simulink model "FBsimDC_closed"  (R2018b)
settings: Solver=ode4  StartTime=0.0  StopTime=0.5e-3*0+0.5*1+0.8*0  FixedStep=Tsim  MaxStep=1e-4  RelTol=1e-6
PreLoadFcn:
  | uC=Simulink.Signal;
  | uC.RTWInfo.STorageClass='ExportedGlobal';
  | uC.InitialValue='0.5';
undefined symbols (not defined in the file): C1, C3, fsw, imax, J, Ke, kiI, kiMR, kiW, kpI, kpMR, kpW, Kt, La, Ra, Ts, Tsim, Tsm, Tw, Vdc, wmax
libraries: powerlib x11, simulink x7, powerlib_meascontrol x1, peGeneralControl x1
settings Model: Creator=matti  LastModifiedBy=matti
settings DataIOCC: ReturnWorkspaceOutputs=on

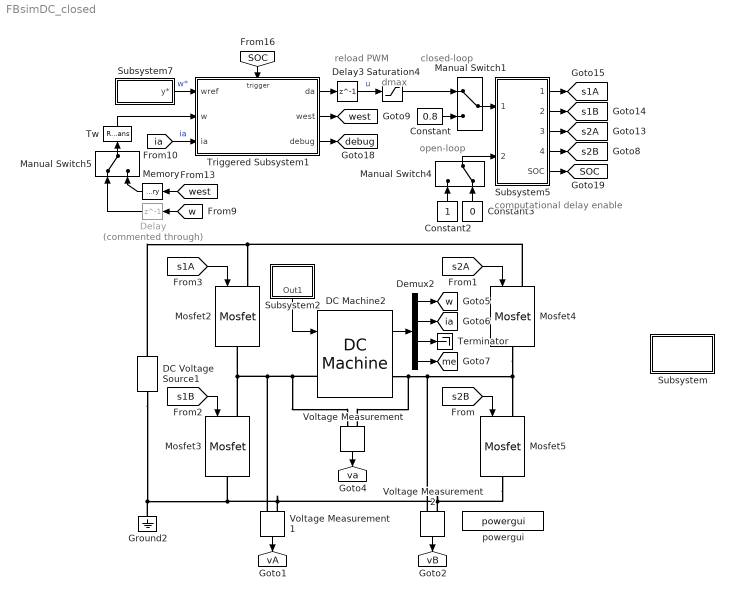
== system FBsimDC_closed ==
  note: closed-loop
  note: open-loop
  note: reload
      | PWM
  note: computational delay
      | enable
  note: dmax
  Constant : Constant  Value=0.8  SampleTime=Ts
  Constant2 : Constant  SampleTime=Ts
  Constant3 : Constant  Value=0  SampleTime=Ts
  DC Machine2 : powerlib/Machines/DC Machine  PresetModel=No  MechanicalLoad=Torque TL  FieldType=Permanent magnet  ShowDetailedParameters=on  MeasurementBus=off  RLa="[Ra  La]"  RLf="[ 240  120]"  Laf=1.8  MachineConstant=Torque constant (N.m/A)  Ke=1.8  Kt=Kt  J=J  Bm=B  Tf=0  w0=0  Ifinit=1  TsPowergui=0  TsBlock=-1
      settings: SourceProductName=Simscape Electrical
  DC Voltage Source1 : powerlib/Electrical Sources/DC Voltage Source  Amplitude=Vdc  Measurements=None
      settings: SourceProductName=Simscape Electrical
  Delay : Delay  Commented=through  DelayLength=1  SampleTime=Tw
  Delay3 : Delay  DelayLength=1  InitialCondition=0.5  SampleTime=Ts/2
  Demux2 : Demux  BusSelectionMode=on
  Ground2 : powerlib/Elements/Ground  LConnTagsString=a
      settings: SourceProductName=Simscape Electrical
  Manual Switch1 : ManualSwitch
  Manual Switch4 : ManualSwitch  CurrentSetting=0
  Manual Switch5 : ManualSwitch
  Memory : Memory  InheritSampleTime=on
  Mosfet{2..5} (4 alike) : powerlib/Power Electronics/Mosfet  Ron=0.1  Lon=0  Rd=0.01  Vfd=0  IC=0  Rs=1e5  Cs=inf  Measurements=off
      settings: SourceProductName=Simscape Electrical
  Saturation4 : Saturate  UpperLimit=1  LowerLimit=0
  Subsystem : Subsystem
      mask Display: disp('stream')
  Subsystem2 : Subsystem
      mask Display: disp('load\ntorque')
  Subsystem5 : Subsystem
      mask Display: disp('modulator')
  Subsystem7 : Subsystem
      mask Display: disp('reference')
  Terminator : Terminator
  Triggered Subsystem1 : Subsystem  TreatAsAtomicUnit=on
      mask Display: disp('cascade controller\n(syncronized with PWM)')
  Tw : RateTransition  OutPortSampleTime=Tw
  Voltage Measurement : powerlib/Measurements/Voltage Measurement  PhasorSimulation=off  OutputType=Complex  PSBequivalent=0
  Voltage Measurement1 : powerlib/Measurements/Voltage Measurement  PhasorSimulation=off  OutputType=Complex  PSBequivalent=0
  Voltage Measurement2 : powerlib/Measurements/Voltage Measurement  PhasorSimulation=off  OutputType=Complex  PSBequivalent=0
  powergui : powerlib/powergui  Priority=1  SimulationMode=Continuous  SampleTime=1/(400*fsw)  frequency=60  Iterations=50  frequencyindice=0  Pbase=100e6  ErrMax=1e-4  UnitsV=kV  UnitsW=MW  buscounter=0  FunctionMessages=on  echomessages=off  EnableUseOfTLC=off  CurrentSourceSwitches=off  DisableSnubberDevices=on  DisableRonSwitches=on  DisableVfSwitches=on  DisplayEquations=off  SolverType=Tustin/Backward Euler (TBE)  Interpol=off  ExternalGateDelay=off  methode=off  Ts=100  x0status=blocks  SPID=off  SwTol=0  HookPort=off  RestoreLinks=warning  ResistiveCurrentMeasurement=off  Frange=[0:2:500]  Ylog=off  Xlog=on  ShowGrid=off  save=off  variable=ZData  structure=0  ZoomFFT=off  StartTime=0.0  cycles=1  DisplayStyle=1  fundamental=60  FreqAxis=off  MaxFrequency=1000  frequencyindicesteady=1  RmsSteady=1  display=off
  tag scope: SOC=global, debug=global, ia=global, me=global, s1A=global, s1B=global, s2A=global, s2B=global, vA=global, vB=global, va=global, w=global, west=global
  wires:
  DC Machine2/1 -> Demux2/1
  [s2B] -> Mosfet5/1
  [s2A] -> Mosfet4/1
  [s1B] -> Mosfet3/1
  [s1A] -> Mosfet2/1
  Demux2/3 -> Terminator/1
  Voltage Measurement/1 -> [va]
  Demux2/1 -> [w]
  Demux2/2 -> [ia]
  Demux2/4 -> [me]
  Subsystem5/3(Out3) -> [s2A]
  Subsystem5/1(Out1) -> [s1A]
  Subsystem5/4(Out4) -> [s2B]
  Subsystem5/2(Out2) -> [s1B]
  Manual Switch1/1 -> Subsystem5/1(modA)
  Saturation4/1 -> Manual Switch1/1
  Constant/1 -> Manual Switch1/2
  Subsystem2/1(Out1) -> DC Machine2/1
  [west] -> Memory/1
  Triggered Subsystem1/1(da) -> Delay3/1
  Manual Switch5/1 -> Tw/1
  [SOC] -> Triggered Subsystem1/Trigger
  Constant3/1 -> Manual Switch4/2
  Subsystem7/1(y*) -> Triggered Subsystem1/1(wref)  "w*"
  Delay3/1 -> Saturation4/1  "u"
  Triggered Subsystem1/3(debug) -> [debug]
  Constant2/1 -> Manual Switch4/1
  Manual Switch4/1 -> Subsystem5/2(enable delay)
  Subsystem5/5(SOC) -> [SOC]
  [ia] -> Triggered Subsystem1/3(ia)  "ia"
  Triggered Subsystem1/2(west) -> [west]
  Memory/1 -> Manual Switch5/2
  Voltage Measurement1/1 -> [vA]
  Voltage Measurement2/1 -> [vB]
  Tw/1 -> Triggered Subsystem1/2(w)
  [w] -> Delay/1
  Delay/1 -> Manual Switch5/1
  connections:
  Mosfet3/RConn1 -- Voltage Measurement2/LConn2 -- Mosfet5/RConn1 -- Voltage Measurement1/LConn2 -- Ground2/LConn1 -- DC Voltage Source1/LConn1
  Mosfet4/LConn1 -- DC Voltage Source1/RConn1 -- Mosfet2/LConn1
  Mosfet4/RConn1 -- Voltage Measurement2/LConn1 -- Voltage Measurement/LConn2 -- DC Machine2/RConn1 -- Mosfet5/LConn1
  Mosfet3/LConn1 -- Voltage Measurement1/LConn1 -- DC Machine2/LConn1 -- Voltage Measurement/LConn1 -- Mosfet2/RConn1

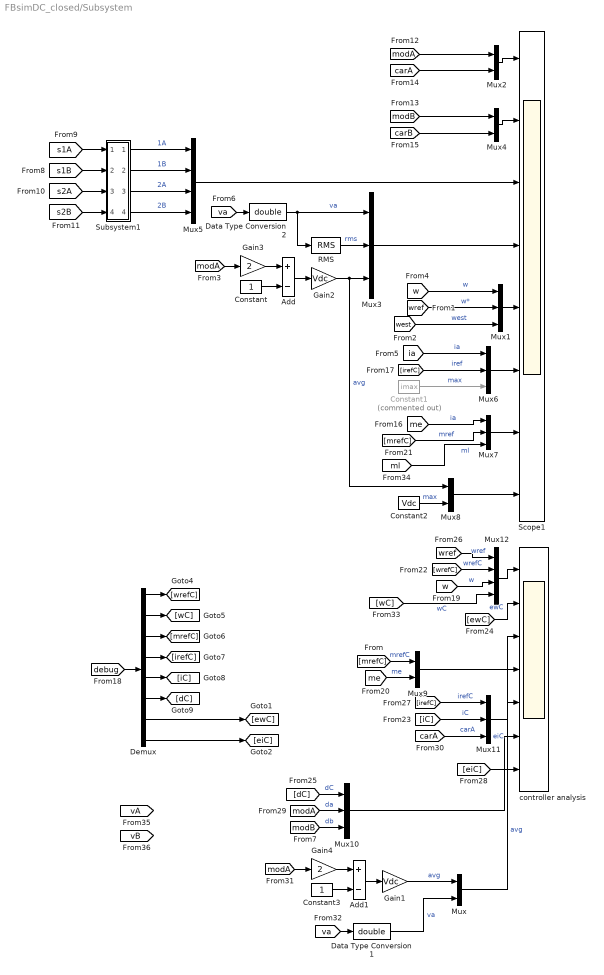
== system FBsimDC_closed/Subsystem ==
  Add : Sum  Inputs=+-
  Add1 : Sum  Inputs=+-
  Constant : Constant  SampleTime=Ts
  Constant1 : Constant  Commented=on  Value=imax  SampleTime=Ts
  Constant2 : Constant  Value=Vdc  SampleTime=Ts
  Constant3 : Constant  SampleTime=Ts
  Data Type Conversion1 : DataTypeConversion  OutDataTypeStr=double
  Data Type Conversion2 : DataTypeConversion  OutDataTypeStr=double
  Demux : Demux  Outputs=8
  Gain1 : Gain  Gain=Vdc
  Gain2 : Gain  Gain=Vdc
  Gain3 : Gain  Gain=2
  Gain4 : Gain  Gain=2
  Mux{,2,4,8..9} (5 alike) : Mux  Inputs=2
  Mux{1,3,6..7,10..11} (6 alike) : Mux  Inputs=3
  Mux12 : Mux
  Mux5 : Mux
  RMS : powerlib_meascontrol/Measurements/RMS  TrueRMS=on  Freq=fsw  RMSInit=0  Ts=0
  Scope1 : Scope  NumInputPorts=8
  Subsystem1 : Subsystem
      mask Display: disp('shift')
  controller analysis : Scope  NumInputPorts=7
  wires:
  [modA] -> Mux2/1
  Mux3/1 -> Scope1/4
  [s2B] -> Subsystem1/4(In4)
  [carA] -> Mux2/2
  [s1A] -> Subsystem1/1(In1)
  [va] -> Data Type Conversion2/1
  Mux2/1 -> Scope1/1
  [s2A] -> Subsystem1/3(In3)
  Mux4/1 -> Scope1/2
  [modB] -> Mux4/1
  Data Type Conversion2/1 -> Mux3/1, RMS/1  "va"
  [s1B] -> Subsystem1/2(In2)
  [carB] -> Mux4/2
  Subsystem1/3(Out3) -> Mux5/3  "2A"
  Subsystem1/4(Out4) -> Mux5/4  "2B"
  Subsystem1/2(Out2) -> Mux5/2  "1B"
  Subsystem1/1(Out1) -> Mux5/1  "1A"
  Mux5/1 -> Scope1/3
  Gain3/1 -> Add/1
  Gain2/1 -> Mux3/3, Mux8/1  "avg"
  Constant/1 -> Add/2
  [modA] -> Gain3/1
  Add/1 -> Gain2/1
  RMS/1 -> Mux3/2  "rms"
  [irefC] -> Mux6/2  "iref"
  [ia] -> Mux6/1  "ia"
  Mux6/1 -> Scope1/6
  [wref] -> Mux1/2  "w*"
  [w] -> Mux1/1  "w"
  Mux1/1 -> Scope1/5
  Mux7/1 -> Scope1/7
  [me] -> Mux7/1  "ia"
  [mrefC] -> Mux7/2  "mref"
  Constant1/1 -> Mux6/3  "max"
  Mux8/1 -> Scope1/8
  Constant2/1 -> Mux8/2  "max"
  [west] -> Mux1/3  "west"
  [debug] -> Demux/1
  Mux11/1 -> controller analysis/4
  [carA] -> Mux11/3  "carA"
  [dC] -> Mux10/1  "dC"
  [wrefC] -> Mux12/2  "wrefC"
  [modA] -> Mux10/2  "da"
  [irefC] -> Mux11/1  "irefC"
  Mux12/1 -> controller analysis/1
  [iC] -> Mux11/2  "iC"
  [wref] -> Mux12/1  "wref"
  Mux10/1 -> controller analysis/6
  Demux/1 -> [wrefC]
  Demux/2 -> [wC]
  Demux/3 -> [mrefC]
  Demux/4 -> [irefC]
  Demux/5 -> [iC]
  Demux/6 -> [dC]
  [w] -> Mux12/3  "w"
  Mux9/1 -> controller analysis/3
  [mrefC] -> Mux9/1  "mrefC"
  [me] -> Mux9/2  "me"
  [modB] -> Mux10/3  "db"
  [ewC] -> controller analysis/2  "ewC"
  Demux/7 -> [ewC]
  Demux/8 -> [eiC]
  [eiC] -> controller analysis/5  "eiC"
  Add1/1 -> Gain1/1
  [modA] -> Gain4/1
  Constant3/1 -> Add1/2
  Gain4/1 -> Add1/1
  Mux/1 -> controller analysis/7  "avg"
  [va] -> Data Type Conversion1/1
  Gain1/1 -> Mux/1  "avg"
  Data Type Conversion1/1 -> Mux/2  "va"
  [wC] -> Mux12/4  "wC"
  [ml] -> Mux7/3  "ml"

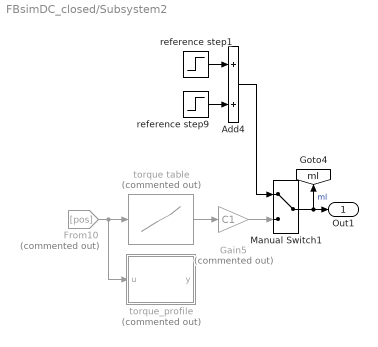
== system FBsimDC_closed/Subsystem2 ==
  Add4 : Sum
  From10 : From  Commented=on  GotoTag=pos  TagVisibility=global
  Gain5 : Gain  Commented=on  Gain=C1
  Manual Switch1 : ManualSwitch
  reference step1 : Step  Time=0.1  After=0.03  SampleTime=Ts
  reference step9 : Step  Time=0.3  After=-0.03  SampleTime=Ts
  torque table : Lookup_n-D  Commented=on  NumberOfTableDimensions=1  BreakpointsForDimension1=[0 1 3 4 6 8 9 10]  Table=[ 0, 0, 26000*9.81*sin(atan(5/100)), 0, 0, 26000*9.81*sin(atan(-5/100)), 0 0]  InterpMethod=Flat  InternalRulePriority=Speed  RndMeth=Simplest  InputSameDT=on
  torque_profile : MATLAB Function  Commented=on  TreatAsAtomicUnit=on
  Out1 : Outport
  tag scope: ml=global
  wires:
  Manual Switch1/1 -> [ml], Out1/1  "ml"
  torque table/1 -> Gain5/1
  From10/1 -> torque_profile/1(u), torque table/1
  Gain5/1 -> Manual Switch1/2
  reference step9/1 -> Add4/2
  Add4/1 -> Manual Switch1/1
  reference step1/1 -> Add4/1

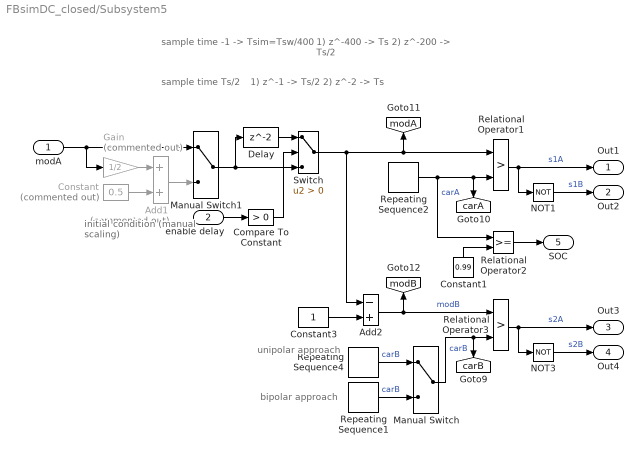
== system FBsimDC_closed/Subsystem5 ==
  note: initial condition
      | (manual scaling)
  note: unipolar approach
  note: bipolar approach
  note: sample time Ts/2
  note: sample time -1 -> Tsim=Tsw/400
  note: 1)  z^-1 -> Ts/2
      | 2)  z^-2 -> Ts
  note: 1)  z^-400 -> Ts
      | 2)  z^-200 -> Ts/2
  modA : Inport
  enable delay : Inport  Port=2
  Add1 : Sum  Commented=on
  Add2 : Sum  Inputs=-+
  Compare To Constant : simulink/Logic and Bit Operations/Compare To Constant  relop=>  const=0  OutDataTypeStr=boolean
  Constant : Constant  Commented=on  Value=0.5  SampleTime=Ts
  Constant1 : Constant  Value=0.99  SampleTime=Ts
  Constant3 : Constant  SampleTime=Ts
  Delay : Delay  SampleTime=Ts
  Gain : Gain  Commented=on  Gain=1/2
  Manual Switch : ManualSwitch
  Manual Switch1 : ManualSwitch
  NOT1 : Logic  Operator=NOT  IconShape=distinctive  AllPortsSameDT=off  OutDataTypeStr=boolean
  NOT3 : Logic  Operator=NOT  IconShape=distinctive  AllPortsSameDT=off  OutDataTypeStr=boolean
  Relational Operator1 : RelationalOperator  Operator=>  OutDataTypeStr=boolean  RndMeth=Simplest
  Relational Operator2 : RelationalOperator  OutDataTypeStr=boolean  RndMeth=Simplest
  Relational Operator3 : RelationalOperator  Operator=>  OutDataTypeStr=boolean  RndMeth=Simplest
  Repeating Sequence1 : simulink/Sources/Repeating Sequence  rep_seq_t=[0 1/(2*fsw) 1/fsw]  rep_seq_y=[1 0 1]
  Repeating Sequence2 : simulink/Sources/Repeating Sequence  rep_seq_t=[0 1/(2*fsw) 1/fsw]  rep_seq_y=[0 1 0]
  Repeating Sequence4 : simulink/Sources/Repeating Sequence  rep_seq_t=[0 1/(2*fsw) 1/fsw]  rep_seq_y=[0 1 0]
  Switch : Switch  Criteria=u2 > Threshold
  Out1 : Outport
  Out2 : Outport  Port=2
  Out3 : Outport  Port=3
  Out4 : Outport  Port=4
  SOC : Outport  Port=5
  tag scope: carA=global, carB=global, modA=global, modB=global
  wires:
  Constant3/1 -> Add2/2
  Manual Switch/1 -> [carB], Relational Operator3/2  "carB"
  Add2/1 -> Relational Operator3/1, [modB]  "modB"
  Relational Operator3/1 -> Out3/1, NOT3/1  "s2A"
  Repeating Sequence1/1 -> Manual Switch/2  "carB"
  NOT3/1 -> Out4/1  "s2B"
  Repeating Sequence4/1 -> Manual Switch/1  "carB"
  Relational Operator1/1 -> Out1/1, NOT1/1  "s1A"
  NOT1/1 -> Out2/1  "s1B"
  modA/1 -> Manual Switch1/1, Gain/1
  Constant/1 -> Add1/2
  Add1/1 -> Manual Switch1/2
  Gain/1 -> Add1/1
  Relational Operator2/1 -> SOC/1
  Repeating Sequence2/1 -> Relational Operator2/1, [carA], Relational Operator1/2  "carA"
  Constant1/1 -> Relational Operator2/2
  Switch/1 -> Add2/1, Relational Operator1/1, [modA]
  Compare To Constant/1 -> Switch/2
  Delay/1 -> Switch/1
  enable delay/1 -> Compare To Constant/1
  Manual Switch1/1 -> Delay/1, Switch/3

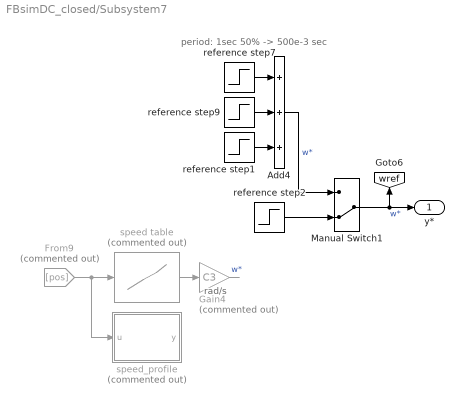
== system FBsimDC_closed/Subsystem7 ==
  note: period: 1sec 50% -> 500e-3 sec
  note: rad/s
  Add4 : Sum  Inputs=+++
  From9 : From  Commented=on  GotoTag=pos
  Gain4 : Gain  Commented=on  Gain=C3
  Manual Switch1 : ManualSwitch  CurrentSetting=0
  reference step1 : Step  Time=0.005+0.15+500e-3  After=200  SampleTime=Ts
  reference step2 : Step  Time=0.005  After=100  SampleTime=Ts
  reference step7 : Step  Time=0.005  After=100  SampleTime=Ts
  reference step9 : Step  Time=0.005+0.15  After=-200  SampleTime=Ts
  speed table : Lookup_n-D  Commented=on  NumberOfTableDimensions=1  BreakpointsForDimension1=[0 1 3 4 6 8 9 10]  Table=[35 60 60 75 60 60 35 0]  InterpMethod=Flat  ExtrapMethod=Clip  UseLastTableValue=on  InternalRulePriority=Speed  RndMeth=Simplest  InputSameDT=on
  speed_profile : MATLAB Function  Commented=on  TreatAsAtomicUnit=on
  y* : Outport
  tag scope: wref=global
  wires:
  Manual Switch1/1 -> [wref], y*/1  "w*"
  Add4/1 -> Manual Switch1/1  "w*"
  From9/1 -> speed_profile/1(u), speed table/1
  speed table/1 -> Gain4/1
  Gain4/1 -> ?  "w*"
  reference step7/1 -> Add4/1
  reference step9/1 -> Add4/2
  reference step1/1 -> Add4/3
  reference step2/1 -> Manual Switch1/2

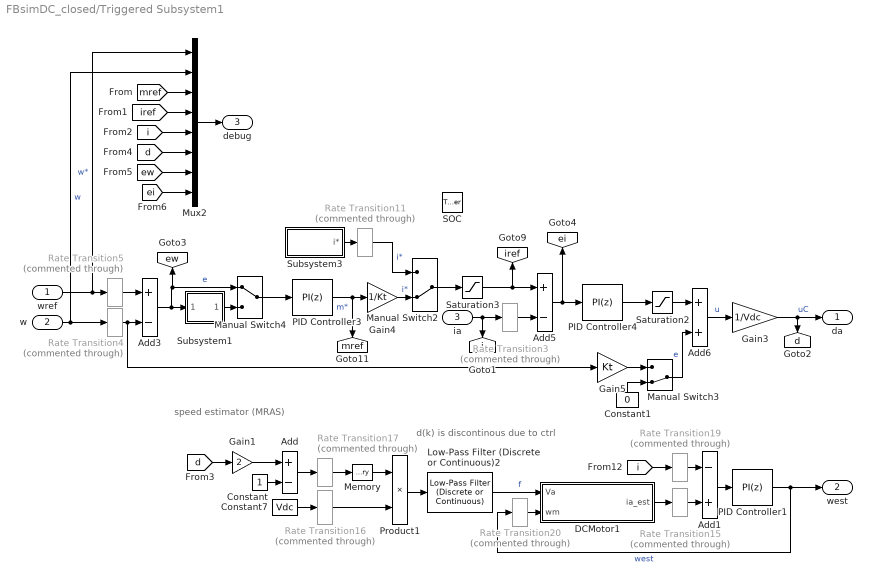
== system FBsimDC_closed/Triggered Subsystem1 ==
  note: d(k) is discontinous
      | due to ctrl
  note: speed estimator (MRAS)
  wref : Inport
  w : Inport  Port=2
  ia : Inport  Port=3
  SOC : TriggerPort  VariantControl=Variant
  Add : Sum  Inputs=+-
  Add1 : Sum  Inputs=-+
  Add3 : Sum  Inputs=+-
  Add5 : Sum  Inputs=+-
  Add6 : Sum
  Constant : Constant  SampleTime=-1
  Constant1 : Constant  Value=0  SampleTime=-1
  Constant7 : Constant  Value=Vdc  SampleTime=-1
  DCMotor1 : Subsystem
      mask Display:
      | disp('Adaptive\nmodel')
      | port_label('input', 1, 'va')
      | port_label('input', 2, 'wm')
      | port_label('output', 1, 'ia est.')
  Gain1 : Gain  Gain=2
  Gain3 : Gain  Gain=1/Vdc
  Gain4 : Gain  Gain=1/Kt
  Gain5 : Gain  Gain=Kt
  Low-Pass Filter (Discrete or Continuous)2 : peGeneralControl/Low-Pass Filter (Discrete or Continuous)  K=1  T=0.0008  B=20  A=-20  Ts=-1
  Manual Switch2 : ManualSwitch  CurrentSetting=0
  Manual Switch3 : ManualSwitch  CurrentSetting=0
  Manual Switch4 : ManualSwitch
  Memory : Memory  InheritSampleTime=on
  Mux2 : Mux  Inputs=8
  PID Controller1 : simulink/Continuous/PID Controller  Controller=PI  Form=Parallel  TimeDomain=Discrete-time  SampleTime=-1  IntegratorMethod=Forward Euler  FilterMethod=Forward Euler  ControllerParametersSource=internal  P=kpMR  I=kiMR  D=kiMR*5  UseFilter=on  N=100  TunerSelectOption=Transfer Function Based (PID Tuner App)  ZeroCross=off  InitialConditionSource=internal  InitialConditionForIntegrator=0  InitialConditionForFilter=0  DifferentiatorICPrevScaledInput=0  ExternalReset=none  TrackingMode=off  Kt=1  LimitOutput=on  UpperSaturationLimit=wmax  LowerSaturationLimit=-wmax  LinearizeAsGain=off  AntiWindupMode=back-calculation  Kb=kiMR/kpMR  POutMin=[]  POutMax=[]  IOutMin=[]  IOutMax=[]  DOutMin=[]  DOutMax=[]  NOutMin=[]  NOutMax=[]  SumOutMin=[]  SumOutMax=[]  SaturationOutMin=[]  SaturationOutMax=[]  PParamMin=[]  PParamMax=[]  IParamMin=[]  IParamMax=[]  DParamMin=[]  DParamMax=[]  NParamMin=[]  NParamMax=[]  KbParamMin=[]  KbParamMax=[]  KtParamMin=[]  KtParamMax=[]  KbOutMin=[]  KbOutMax=[]  KtOutMin=[]  KtOutMax=[]  IntegratorOutMin=[]  IntegratorOutMax=[]  FilterOutMin=[]  FilterOutMax=[]  SumI1OutMin=[]  SumI1OutMax=[]  SumI2OutMin=[]  SumI2OutMax=[]  SumI3OutMin=[]  SumI3OutMax=[]  SumI4OutMin=[]  SumI4OutMax=[]  SumDOutMin=[]  SumDOutMax=[]  DifferentiatorOutMin=[]  DifferentiatorOutMax=[]  FilterDiffOutCoefMin=[]  FilterDiffOutCoefMax=[]  ReciprocalOutMin=[]  ReciprocalOutMax=[]  SumDenOutMin=[]  SumDenOutMax=[]  SumNumOutMin=[]  SumNumOutMax=[]  DivideOutMin=[]  DivideOutMax=[]  IntegratorContinuousStateAttributes=''  IntegratorStateMustResolveToSignalObject=off  IntegratorRTWStateStorageClass=Auto  FilterContinuousStateAttributes=''  FilterStateMustResolveToSignalObject=off  FilterRTWStateStorageClass=Auto  ParallelPVariant=InternalParameters  IdealPVariant=Disabled  IVariant=InternalParameters  DVariant=Disabled  IntegratorVariant=Discrete  SatVariant=Enabled  AWVariant=BackCalculation  PCopyVariant=Disabled  TRVariant=Disabled  FdbkBlocksVariant=Forward  IdealPFdbkVariant=Disabled  SatFdbkVariant=Disabled  DerivativeFilterVariant=Disabled  NVariant=Disabled  NCopyVariant=Disabled_SignalSpec  FilterICVariant=Disabled  IntegratorICVariant=InternalICs  ExternalResetVariant=Disabled  TRSumVariant=Passthrough  SumFdbkVariant=Disabled  SumVariant=Sum_PI
  PID Controller3 : simulink/Continuous/PID Controller  Controller=PI  Form=Parallel  TimeDomain=Discrete-time  SampleTime=-1  IntegratorMethod=Forward Euler  FilterMethod=Forward Euler  ControllerParametersSource=internal  P=kpW  I=kiW  D=0  UseFilter=on  N=100  TunerSelectOption=Transfer Function Based (PID Tuner App)  InitialConditionSource=internal  InitialConditionForIntegrator=0  InitialConditionForFilter=0  DifferentiatorICPrevScaledInput=0  ExternalReset=none  TrackingMode=off  Kt=1  LimitOutput=on  UpperSaturationLimit=Kt*imax  LowerSaturationLimit=-Kt*imax  LinearizeAsGain=off  AntiWindupMode=back-calculation  Kb=kiW/kpW  POutMin=[]  POutMax=[]  IOutMin=[]  IOutMax=[]  DOutMin=[]  DOutMax=[]  NOutMin=[]  NOutMax=[]  SumOutMin=[]  SumOutMax=[]  SaturationOutMin=[]  SaturationOutMax=[]  PParamMin=[]  PParamMax=[]  IParamMin=[]  IParamMax=[]  DParamMin=[]  DParamMax=[]  NParamMin=[]  NParamMax=[]  KbParamMin=[]  KbParamMax=[]  KtParamMin=[]  KtParamMax=[]  KbOutMin=[]  KbOutMax=[]  KtOutMin=[]  KtOutMax=[]  IntegratorOutMin=[]  IntegratorOutMax=[]  FilterOutMin=[]  FilterOutMax=[]  SumI1OutMin=[]  SumI1OutMax=[]  SumI2OutMin=[]  SumI2OutMax=[]  SumI3OutMin=[]  SumI3OutMax=[]  SumI4OutMin=[]  SumI4OutMax=[]  SumDOutMin=[]  SumDOutMax=[]  DifferentiatorOutMin=[]  DifferentiatorOutMax=[]  FilterDiffOutCoefMin=[]  FilterDiffOutCoefMax=[]  ReciprocalOutMin=[]  ReciprocalOutMax=[]  SumDenOutMin=[]  SumDenOutMax=[]  SumNumOutMin=[]  SumNumOutMax=[]  DivideOutMin=[]  DivideOutMax=[]  IntegratorContinuousStateAttributes=''  IntegratorStateMustResolveToSignalObject=off  IntegratorRTWStateStorageClass=Auto  FilterContinuousStateAttributes=''  FilterStateMustResolveToSignalObject=off  FilterRTWStateStorageClass=Auto  ParallelPVariant=InternalParameters  IdealPVariant=Disabled  IVariant=InternalParameters  DVariant=Disabled  IntegratorVariant=Discrete  SatVariant=Enabled  AWVariant=BackCalculation  PCopyVariant=Disabled  TRVariant=Disabled  FdbkBlocksVariant=Forward  IdealPFdbkVariant=Disabled  SatFdbkVariant=Disabled  DerivativeFilterVariant=Disabled  NVariant=Disabled  NCopyVariant=Disabled_SignalSpec  FilterICVariant=Disabled  IntegratorICVariant=InternalICs  ExternalResetVariant=Disabled  TRSumVariant=Passthrough  SumFdbkVariant=Disabled  SumVariant=Sum_PI
  PID Controller4 : simulink/Continuous/PID Controller  Controller=PI  Form=Parallel  TimeDomain=Discrete-time  SampleTime=-1  IntegratorMethod=Forward Euler  FilterMethod=Forward Euler  ControllerParametersSource=internal  P=kpI  I=kiI  D=0  UseFilter=on  N=100  TunerSelectOption=Transfer Function Based (PID Tuner App)  InitialConditionSource=internal  InitialConditionForIntegrator=Vdc/2  InitialConditionForFilter=0  DifferentiatorICPrevScaledInput=0  ExternalReset=none  TrackingMode=off  Kt=1  LimitOutput=on  UpperSaturationLimit=Vdc*0.98  LowerSaturationLimit=0  LinearizeAsGain=off  AntiWindupMode=back-calculation  Kb=kiI/kpI  POutMin=[]  POutMax=[]  IOutMin=[]  IOutMax=[]  DOutMin=[]  DOutMax=[]  NOutMin=[]  NOutMax=[]  SumOutMin=[]  SumOutMax=[]  SaturationOutMin=[]  SaturationOutMax=[]  PParamMin=[]  PParamMax=[]  IParamMin=[]  IParamMax=[]  DParamMin=[]  DParamMax=[]  NParamMin=[]  NParamMax=[]  KbParamMin=[]  KbParamMax=[]  KtParamMin=[]  KtParamMax=[]  KbOutMin=[]  KbOutMax=[]  KtOutMin=[]  KtOutMax=[]  IntegratorOutMin=[]  IntegratorOutMax=[]  FilterOutMin=[]  FilterOutMax=[]  SumI1OutMin=[]  SumI1OutMax=[]  SumI2OutMin=[]  SumI2OutMax=[]  SumI3OutMin=[]  SumI3OutMax=[]  SumI4OutMin=[]  SumI4OutMax=[]  SumDOutMin=[]  SumDOutMax=[]  DifferentiatorOutMin=[]  DifferentiatorOutMax=[]  FilterDiffOutCoefMin=[]  FilterDiffOutCoefMax=[]  ReciprocalOutMin=[]  ReciprocalOutMax=[]  SumDenOutMin=[]  SumDenOutMax=[]  SumNumOutMin=[]  SumNumOutMax=[]  DivideOutMin=[]  DivideOutMax=[]  IntegratorContinuousStateAttributes=''  IntegratorStateMustResolveToSignalObject=off  IntegratorRTWStateStorageClass=Auto  FilterContinuousStateAttributes=''  FilterStateMustResolveToSignalObject=off  FilterRTWStateStorageClass=Auto  ParallelPVariant=InternalParameters  IdealPVariant=Disabled  IVariant=InternalParameters  DVariant=Disabled  IntegratorVariant=Discrete  SatVariant=Enabled  AWVariant=BackCalculation  PCopyVariant=Disabled  TRVariant=Disabled  FdbkBlocksVariant=Forward  IdealPFdbkVariant=Disabled  SatFdbkVariant=Disabled  DerivativeFilterVariant=Disabled  NVariant=Disabled  NCopyVariant=Disabled_SignalSpec  FilterICVariant=Disabled  IntegratorICVariant=InternalICs  ExternalResetVariant=Disabled  TRSumVariant=Passthrough  SumFdbkVariant=Disabled  SumVariant=Sum_PI
  Product1 : Product
  Rate Transition{3..5,11} (4 alike) : RateTransition  Commented=through  Integrity=off  OutPortSampleTime=Ts
  Rate Transition{15..17,19..20} (5 alike) : RateTransition  Commented=through  Integrity=off  OutPortSampleTime=Tsm
  Saturation2 : Saturate  UpperLimit=Vdc  LowerLimit=0
  Saturation3 : Saturate  UpperLimit=imax  LowerLimit=-imax
  Subsystem1 : Subsystem
      mask Display: disp('cut\nnoise')
  Subsystem3 : Subsystem
      mask Display: disp('reference')
  da : Outport  InitialOutput=[0.5]
  west : Outport  Port=2
  debug : Outport  Port=3
  tag scope: d=global, ei=global, ew=global, i=global, iref=global, mref=global
  wires:
  Gain3/1 -> da/1, [d]  "uC"
  ia/1 -> [i], Rate Transition3/1
  wref/1 -> Mux2/1, Rate Transition5/1  "w*"
  w/1 -> Mux2/2, Rate Transition4/1  "w"
  PID Controller4/1 -> Saturation2/1
  Gain4/1 -> Manual Switch2/2  "i*"
  Subsystem3/1(i*) -> Rate Transition11/1
  Manual Switch3/1 -> Add6/2  "e"
  Saturation2/1 -> Add6/1
  PID Controller3/1 -> Gain4/1, [mref]  "m*"
  Manual Switch2/1 -> Saturation3/1
  Rate Transition11/1 -> Manual Switch2/1  "i*"
  Gain5/1 -> Manual Switch3/1
  Constant1/1 -> Manual Switch3/2
  Rate Transition5/1 -> Add3/1
  Add6/1 -> Gain3/1  "u"
  Subsystem1/1(Out1) -> Manual Switch4/2
  Add3/1 -> Manual Switch4/1, [ew], Subsystem1/1(In1)  "e"
  Add5/1 -> [ei], PID Controller4/1
  Saturation3/1 -> [iref], Add5/1
  Rate Transition3/1 -> Add5/2
  Rate Transition4/1 -> Gain5/1, Add3/2
  Manual Switch4/1 -> PID Controller3/1
  Mux2/1 -> debug/1
  [mref] -> Mux2/3
  [iref] -> Mux2/4
  [i] -> Mux2/5
  Add1/1 -> PID Controller1/1
  PID Controller1/1 -> west/1, Rate Transition20/1  "west"
  Constant7/1 -> Rate Transition16/1
  [i] -> Rate Transition19/1
  Rate Transition20/1 -> DCMotor1/2(wm)
  Rate Transition15/1 -> Add1/2
  Memory/1 -> Product1/1
  Rate Transition16/1 -> Product1/2
  Product1/1 -> Low-Pass Filter (Discrete or Continuous)2/1
  Rate Transition17/1 -> Memory/1
  DCMotor1/1(ia_est) -> Rate Transition15/1
  Rate Transition19/1 -> Add1/1
  Low-Pass Filter (Discrete or Continuous)2/1 -> DCMotor1/1(Va)  "f"
  [d] -> Mux2/6
  Constant/1 -> Add/2
  [d] -> Gain1/1
  Add/1 -> Rate Transition17/1
  Gain1/1 -> Add/1
  [ew] -> Mux2/7
  [ei] -> Mux2/8

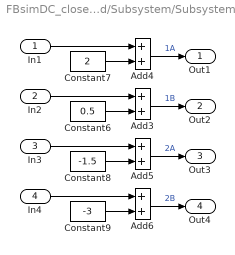
== system FBsimDC_closed/Subsystem/Subsystem1 ==
  In1 : Inport
  In2 : Inport  Port=2
  In3 : Inport  Port=3
  In4 : Inport  Port=4
  Add{3..6} (4 alike) : Sum
  Constant6 : Constant  Value=0.5  SampleTime=Tsim
  Constant7 : Constant  Value=2  SampleTime=Tsim
  Constant8 : Constant  Value=-1.5  SampleTime=Tsim
  Constant9 : Constant  Value=-3  SampleTime=Tsim
  Out1 : Outport
  Out2 : Outport  Port=2
  Out3 : Outport  Port=3
  Out4 : Outport  Port=4
  wires:
  In4/1 -> Add6/1
  In2/1 -> Add3/1
  Constant9/1 -> Add6/2
  In1/1 -> Add4/1
  Constant6/1 -> Add3/2
  Constant8/1 -> Add5/2
  Constant7/1 -> Add4/2
  In3/1 -> Add5/1
  Add4/1 -> Out1/1  "1A"
  Add3/1 -> Out2/1  "1B"
  Add5/1 -> Out3/1  "2A"
  Add6/1 -> Out4/1  "2B"

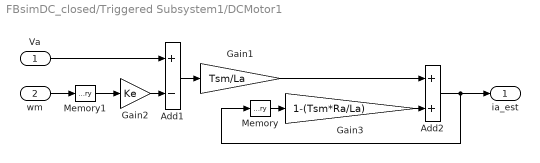
== system FBsimDC_closed/Triggered Subsystem1/DCMotor1 ==
  Va : Inport
  wm : Inport  Port=2
  Add1 : Sum  Inputs=+-
  Add2 : Sum
  Gain1 : Gain  Gain=Tsm/La
  Gain2 : Gain  Gain=Ke
  Gain3 : Gain  Gain=1-(Tsm*Ra/La)
  Memory : Memory  InheritSampleTime=on
  Memory1 : Memory  InheritSampleTime=on
  ia_est : Outport
  wires:
  Gain2/1 -> Add1/2
  wm/1 -> Memory1/1
  Va/1 -> Add1/1
  Add2/1 -> Memory/1, ia_est/1
  Add1/1 -> Gain1/1
  Gain1/1 -> Add2/1
  Gain3/1 -> Add2/2
  Memory/1 -> Gain3/1
  Memory1/1 -> Gain2/1

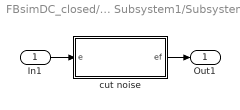
== system FBsimDC_closed/Triggered Subsystem1/Subsystem1 ==
  In1 : Inport
  cut noise : MATLAB Function  TreatAsAtomicUnit=on
  Out1 : Outport
  wires:
  cut noise/1(ef) -> Out1/1
  In1/1 -> cut noise/1(e)

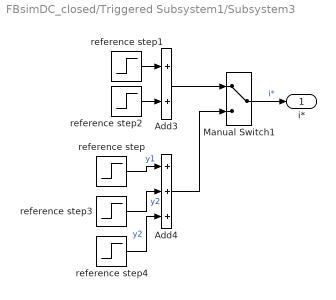
== system FBsimDC_closed/Triggered Subsystem1/Subsystem3 ==
  Add3 : Sum
  Add4 : Sum  Inputs=+++
  Manual Switch1 : ManualSwitch
  reference step : Step  Time=0.02  After=0.4
  reference step1 : Step  Time=0.01
  reference step2 : Step  Time=0.02  After=-1
  reference step3 : Step  Time=0.03  After=-0.8
  reference step4 : Step  Time=0.04  After=0.8
  i* : Outport
  wires:
  Manual Switch1/1 -> i*/1  "i*"
  reference step2/1 -> Add3/2
  Add3/1 -> Manual Switch1/1
  reference step1/1 -> Add3/1
  Add4/1 -> Manual Switch1/2
  reference step/1 -> Add4/1  "y1"
  reference step3/1 -> Add4/2  "y2"
  reference step4/1 -> Add4/3  "y2"

== matlab function FBsimDC_closed/Subsystem2/torque_profile ==
  data: u input; y output
function y = torque_profile(u)
y=0;
if (u>=0 && u<1)
    y=35;
elseif (u>=1 && u<4)
    y=60;
elseif (u>=4 && u<6)
    y=75;
elseif (u>=6 && u<9)
    y=60;
elseif (u>=9 && u<10)
    y=35; 
elseif u>=10
    y=0;
end
end

== matlab function FBsimDC_closed/Subsystem7/speed_profile ==
  data: u input; y output
function y = speed_profile(u)
y=0;
if (u>=0 && u<1)
    y=35;
elseif (u>=1 && u<4)
    y=60;
elseif (u>=4 && u<6)
    y=75;
elseif (u>=6 && u<9)
    y=60;
elseif (u>=9 && u<10)
    y=35; 
elseif u>=10
    y=0;
end
end

== matlab function FBsimDC_closed/Triggered Subsystem1/Subsystem1/cut noise ==
  data: e input; ef output
function ef = cutter(e)
if e <= 0.03 && e >= 0
    ef = 0;
elseif e >= -0.03 && e < 0
    ef = 0;
else
    ef = e;
end
